simulink model "Torquecontrol_2MW"  (R2020a)
settings: Solver=VariableStepAuto  StartTime=0.0  StopTime=120  RelTol=1e-3  EnableMultiTasking=on
values from neighbouring files (symbols this model uses):
  a1 = 0.5176    [data.mat]
  a2 = 116    [data.mat]
  a3 = 0.4    [data.mat]
  a4 = 5    [data.mat]
  a5 = 21    [data.mat]
  a6 = 0.0068    [data.mat]
  a7 = 0.09    [data.mat]
  a8 = 0.035    [data.mat]
  Ad = 6031.85789489    [data.mat]
  denp = den_P    [Wind_Turbine_Pitch.m]    (also in data.mat = [91260000000000 145900000000000 1.431e+17 7.554e+15 2.279e+1)
  dent = den_P    [Wind_Turbine_Pitch.m]    (also in data.mat = [91260000000000 145900000000000 1.431e+17 7.554e+15 2.279e+1)
  nump = num_P    [Wind_Turbine_Pitch.m]    (also in data.mat = [16590000 26450000 25540000000 6335000000 3680000000000])
  numt = num_T    [Wind_Turbine_Pitch.m]    (also in data.mat = [-75000000 -527900000000 -306700000000000])
  sigma = 1 - Lm^2/(Ls*Lr)    (= 0.0661284179513)    [Generator_specs.m]    (also in data.mat = 0.075)
  Tie = 1    [data.mat]
  Tiu = 10000    [data.mat]
  Tix = 1    [data.mat]
  Tpe = 1    [data.mat]
  Tpu = 10000    [data.mat]
  Tpx = 10000    [data.mat]
undefined symbols (not defined in the file or in its folder): sigbuilder_block
settings Model: Creator=likhi  LastModifiedBy=param
settings DataIOCC: ReturnWorkspaceOutputs=off
settings OptimizationCC: LifeSpan=inf
settings DebuggingCC: SFUnexpectedBacktrackingDiag=warning  SFNoUnconditionalDefaultTransitionDiag=warning  SFExecutionAtInitializationDiag=none  ArithmeticOperatorsInVariantConditions=warning
settings SFSimCC: SimUseLocalCustomCode=off  CustomCodeUndefinedFunction=UseInterfaceOnly
settings RTWCC: RTWUseLocalCustomCode=off
settings CodeAppCC: StateflowObjectComments=on
settings GRTTargetCC: TargetLangStandard=C89/C90 (ANSI)
settings ConfigComp: CovMetricSettings=dw  CovHtmlReporting=on  CovSaveCumulativeToWorkspaceVar=on  CovSaveSingleToWorkspaceVar=on  CovExternalEMLEnable=off

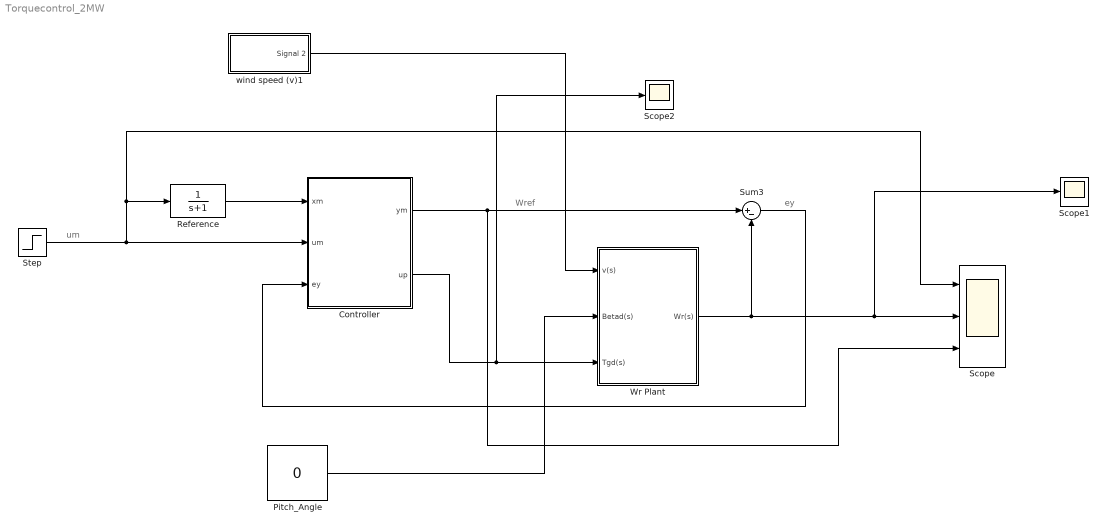
== system Torquecontrol_2MW ==
  note: um
  note: ey
  note: Wref
  Controller : Subsystem
  Pitch_Angle : Constant  Value=0
  Reference : TransferFcn  Denominator=[1 1]
  Scope : Scope  NumInputPorts=3
  Scope1 : Scope
  Scope2 : Scope
  Step : Step  Time=0  After=2  SampleTime=0
  Sum3 : Sum  Inputs=|+-
  Wr Plant : Subsystem
  wind speed (v)1 : Subsystem  Tag=STV Subsys  LoadFcn=sigbuilder_block('load');  StartFcn=sigbuilder_block('start');  StopFcn=sigbuilder_block('stop');  ClipboardFcn=sigbuilder_block('clipboard');  mask(Sigbuilder block){tuvar=[0:10]}
      mask help: Simulink:masks:SigbuilderBlock_MD
      mask init:
      | if ~strcmp(get_param(bdroot(gcbh),'SimulationStatus'),'stopped') tuvar = sigbuilder_block('maskInit'); end
      settings: CopyFcn=sigbuilder_block('copy');  DeleteFcn=sigbuilder_block('delete');  ModelCloseFcn=sigbuilder_block('modelClose');  PreSaveFcn=sigbuilder_block('preSave');  PauseFcn=sigbuilder_block('pause');  ContinueFcn=sigbuilder_block('continue');  NameChangeFcn=sigbuilder_block('namechange');  OpenFcn=sigbuilder_block('open',[6 0 1012.5 477.75 ]);  CloseFcn=sigbuilder_block('close');
      mask Display: plot(0, 0, 100, 100,[2, 2, 32, 32, 2], [68, 8, 8, 68, 68],[32, 2], [38, 38], [32, 19, 2],[53, 60, 44], [32, 17, 17, 2],[16, 16, 31, 31]);txt = getActiveGroup(gcbh);text(2, 100, txt,'verticalAlignment', 'top');
  wires:
  Wr Plant/1(Wr(s)) -> Scope1/1, Scope/2, Sum3/2
  wind speed (v)1/1(Signal 2) -> Wr Plant/1(v(s))
  Sum3/1 -> Controller/3(ey)
  Reference/1 -> Controller/1(xm)
  Step/1 -> Scope/1, Reference/1, Controller/2(um)
  Controller/1(ym) -> Scope/3, Sum3/1
  Pitch_Angle/1 -> Wr Plant/2(Betad(s))
  Controller/2(up) -> Scope2/1, Wr Plant/3(Tgd(s))

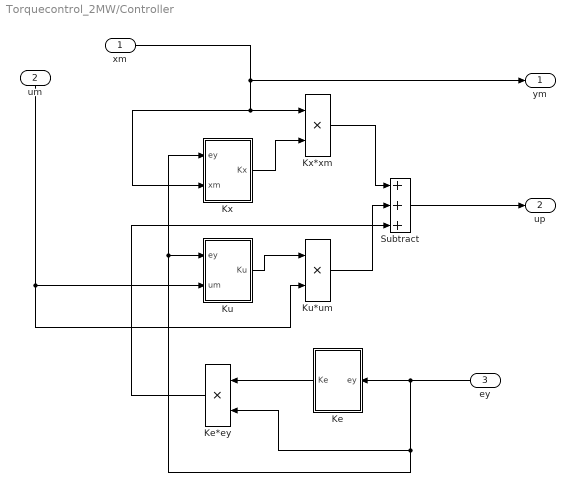
== system Torquecontrol_2MW/Controller ==
  xm : Inport
  um : Inport  Port=2
  ey : Inport  Port=3
  Ke : Subsystem
  Ke*ey : Product
  Ku : Subsystem
  Ku*um : Product
  Kx : Subsystem
  Kx*xm : Product
  Subtract : Sum  Inputs=+++
  ym : Outport
  up : Outport  Port=2
  wires:
  Kx/1(Kx) -> Kx*xm/2
  Ke/1(Ke) -> Ke*ey/1
  Ku*um/1 -> Subtract/2
  Kx*xm/1 -> Subtract/1
  xm/1 -> Kx*xm/1, Kx/2(xm), ym/1
  ey/1 -> Kx/1(ey), Ku/1(ey), Ke*ey/2, Ke/1(ey)
  Ku/1(Ku) -> Ku*um/1
  Ke*ey/1 -> Subtract/3
  um/1 -> Ku/2(um), Ku*um/2
  Subtract/1 -> up/1

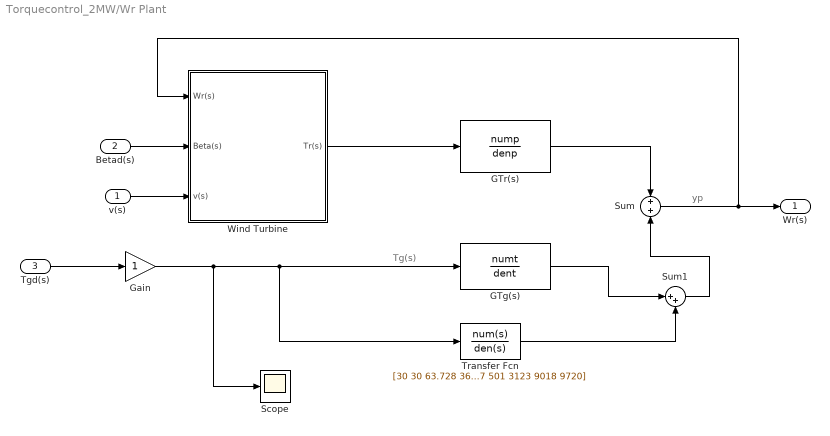
== system Torquecontrol_2MW/Wr Plant ==
  note: yp
  note: Tg(s)
  v(s) : Inport
  Betad(s) : Inport  Port=2
  Tgd(s) : Inport  Port=3
  GTg(s) : TransferFcn  Numerator=numt  Denominator=dent
  GTr(s) : TransferFcn  Numerator=nump  Denominator=denp
  Gain : Gain
  Scope : Scope
  Sum : Sum
  Sum1 : Sum  Inputs=|++
  Transfer Fcn : TransferFcn  Numerator=[30 30 63.728 36.973 30]  Denominator=[1 37 501 3123 9018 9720]
  Wind Turbine : Subsystem  AncestorBlock=re_lib/Wind Generation/Wind Turbine  DialogController=POWERSYS.PowerSysDialog  mask(Wind Turbine){Pnom=2e6, Pelec_base=2e6/0.9, wind_base=9, P_wind_base=0.73, speed_nom=1.2, pitch_angle=0, c1_c6=[0.51763          116          0.4            5           21     0.006795], cp_nom=0.48, lambda_nom=8.1}
      mask prompts: Pnom "Nominal mechanical output power (W):"; Pelec_base "Base power of the electrical generator (VA):"; wind_base "Base wind speed (m/s):"; P_wind_base "Maximum power at base wind speed (pu of nominal mechanical power):"; speed_nom "Base rotational speed (p.u. of base generator speed):"; pitch_angle "Pitch angle beta to display wind-turbine power characteristics (beta >=0)  (deg):"
      mask help:
      | This block implements a variable pitch wind turbine model. The performance coefficient Cp of the turbine is the mechanical output power of the turbine divided by wind power and a function of wind speed, rotational speed, and pitch angle (beta). Cp reaches its maximum value at zero beta. Select the wind-turbine power characteristics display to plot the turbine characteristics at the specified pitch angle.
      |
      | The first input is the generator speed in per unit of the generator base speed. For a synchronous or asynchronous generator, the base speed is the synchronous speed. For a permanent-magnet generator, the base speed is defined as the speed producing nominal voltage at  no load. The second input is the blade pitch angle (beta) in degrees. The third input is the wind speed in m/s.
      |
      | The output is the torque applied to the generator shaft in per unit of the generator ratings.
      |
      | The turbine inertia must be added to the generator inertia.
      mask init:
      | c1=c1_c6(1);c2=c1_c6(2);c3=c1_c6(3);c4=c1_c6(4);c5=c1_c6(5);c6=c1_c6(6);
      | power_initmask();
      mask Help: helpview(psbhelp);
      mask DialogControl DisplayTurbChar Prompt: Display wind turbine power characteristics
      mask DialogControl DisplayTurbChar Callback: WindTurbinePlot(gcb)
      mask Display: disp('');
  Wr(s) : Outport
  wires:
  v(s)/1 -> Wind Turbine/3(v(s))
  Sum/1 -> Wind Turbine/1(Wr(s)), Wr(s)/1
  Tgd(s)/1 -> Gain/1
  GTr(s)/1 -> Sum/1
  Betad(s)/1 -> Wind Turbine/2(Beta(s))
  Wind Turbine/1(Tr(s)) -> GTr(s)/1
  GTg(s)/1 -> Sum1/1
  Transfer Fcn/1 -> Sum1/2
  Sum1/1 -> Sum/2
  Gain/1 -> Scope/1, Transfer Fcn/1, GTg(s)/1

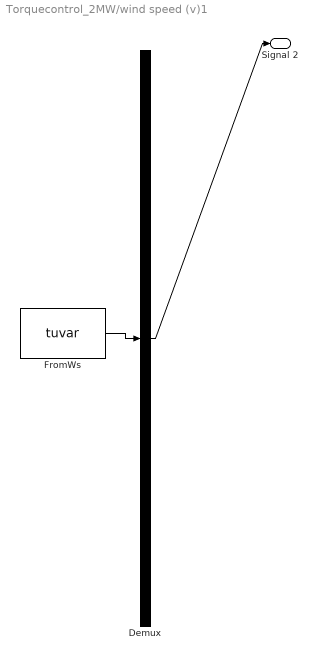
== system Torquecontrol_2MW/wind speed (v)1 ==
  Demux : Demux  Tag=STV Demux  Outputs=1
      settings: DisplayOption=none
  FromWs : FromWorkspace  Tag=STV FromWs  VariableName=tuvar
      SigBuilderData=|
      | common.afterFinalStr = 'Extrapolate'
      | common.sampleTime = 0
      | dataSet(1).timeRange = [0 120]
      | dataSet(1).name = 'Group 1'
      | dataSet(2).timeRange = [0 120]
      | dataSet(2).name = 'Group 2'
      | sbobj.Groups(1).Name = 'Group 1'
      | sbobj.Groups(1).Signals.Name = 'Signal 2'
      | sbobj.Groups(1).Signals.XData = [0 0.1 0.2 0.3 0.4 0.5 0.6 0.7 0.8 0.9 1 1.1 ... (1201 elements, 1x1201)]
      | sbobj.Groups(1).Signals.YData = [15.5376671395 16.8338850146 12.741153139 15.8621733204 15.3187652399 13.6923117037 14.5664079777 15.3426244665 18.5783969397 17.7694370299 13.6501130598 18.0349234663 ... (1201 elements, 1x1201)]
      | sbobj.Groups(1).TimeRange = [0 120]
      | sbobj.Groups(2).Name = 'Group 2'
      | sbobj.Groups(2).Signals.Name = 'Signal 2'
      | sbobj.Groups(2).Signals.XData = [0 1 2 3 4 5 6 7 8 9 10 11 12 13 14 15 16 17 18 19 20 21 22 23 24 25 26 27 28 29 30 31 32 33 34 35 36 37 38 39 40 41 42 43 44 45 46 47 48 49 50 51 52 53 54 55 56 57 58 59 60 61 62 63 64 65 66 67 68 69 70 71 72 73 74 75 76 77 78 79 80 81 82 83 84 85 86 87 88 89 90 91 92 93 94 95 96 97 98 99 100 101 102 103 104 105 106 107 108 109 110 111 112 113 114 115 116 117 118 119 120]
      | sbobj.Groups(2).Signals.YData = [6.01807011575 8.53111911749 8.37266970097 6.38788209314 6.03326297745 6.7836046006 6.68391753827 8.38531742797 6.65170467526 8.20551098078 8.2372434827 9.51972353887 6.62054986454 6.52473145914 8.67572534733 6.26163099795 5.18449703008 7.08672831708 7.50025750546 6.63701916975 6.64930795179 5.63709007085 8.72280393054 7.20137215133 6.45231320782 7.40181236393 7.8343950088 5.95170328812 7.22526321009 6.51763027044 8.65071534952 7.1589257508 5.87531461923 6.88893652325 7.44905097876 9.10058337566 7.03956746808 7.5715725811 8.2007261515 7.50877197187 6.13023828926 6.83893544572 6.34217505374 7.70675183542 8.54031716106 6.97805835356 8.05476174338 6.30324217777 7.15930139 6.82352986481 8.63025921041 7.29396392303 7.76771316613 6.65881339337 6.36659735978 7.39470297405 6.18156140346 5.63827031704 6.69788260596 8.59917448056 6.60767889589 7.22082844093 6.40627813759 4.94960707642 7.00042709296 8.69365989635 6.66847169633 5.84985543786 6.00932777576 7.36418987362 6.57966870551 7.98362168542 6.72423482213 4.91447611455 6.5605287362 7.71192447178 8.02647611247 8.28493457593 8.0007203094 8.07339134627 8.89403249947 8.53443238039 7.17558857287 6.52388222946 6.72025139973 7.70263035474 8.20817483441 6.75244069605 8.51267048749 6.27505286867 6.53466887118 6.61304912341 6.33804960379 7.86990128763 6.81291409702 8.85153725956 6.99387147367 8.86628025483 4.5700315725 7.36181676324 7.28348347922 8.9351889634 7.26172399751 8.77916155129 8.89273585112 6.3796842285 5.80934335084 7.8581940134 6.18492300645 6.8428468059 6.42877121807 7.10081065657 7.59642491901 7.7122037583 7.13564133138 6.05309134985 6.15307228787 7.29230275836 4.8156990126 5.82555531806 5.4342312069]
      | sbobj.Groups(2).TimeRange = [0 120]
  Signal 2 : Outport  Tag=STV Outport
  wires:
  Demux/1 -> Signal 2/1
  FromWs/1 -> Demux/1

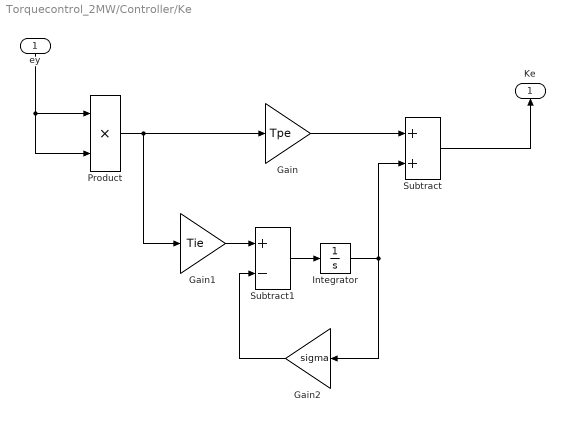
== system Torquecontrol_2MW/Controller/Ke ==
  ey : Inport
  Gain : Gain  Gain=Tpe
  Gain1 : Gain  Gain=Tie
  Gain2 : Gain  Gain=sigma
  Integrator : Integrator
  Product : Product
  Subtract : Sum
  Subtract1 : Sum  Inputs=+-
  Ke : Outport
  wires:
  Subtract/1 -> Ke/1
  ey/1 -> Product/2, Product/1
  Product/1 -> Gain1/1, Gain/1
  Gain/1 -> Subtract/1
  Gain1/1 -> Subtract1/1
  Subtract1/1 -> Integrator/1
  Integrator/1 -> Gain2/1, Subtract/2
  Gain2/1 -> Subtract1/2

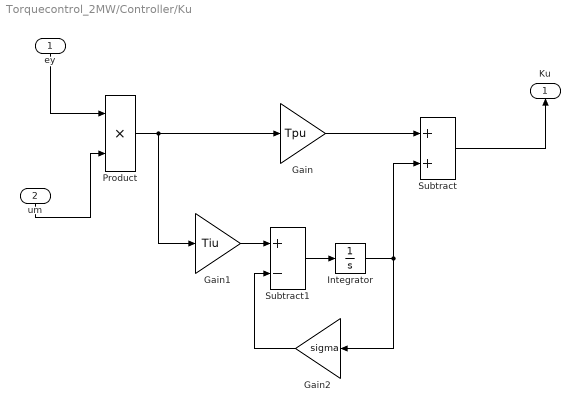
== system Torquecontrol_2MW/Controller/Ku ==
  ey : Inport
  um : Inport  Port=2
  Gain : Gain  Gain=Tpu
  Gain1 : Gain  Gain=Tiu
  Gain2 : Gain  Gain=sigma
  Integrator : Integrator
  Product : Product
  Subtract : Sum
  Subtract1 : Sum  Inputs=+-
  Ku : Outport
  wires:
  Gain2/1 -> Subtract1/2
  Integrator/1 -> Subtract/2, Gain2/1
  Subtract1/1 -> Integrator/1
  Gain1/1 -> Subtract1/1
  Gain/1 -> Subtract/1
  Product/1 -> Gain/1, Gain1/1
  Subtract/1 -> Ku/1
  ey/1 -> Product/1
  um/1 -> Product/2

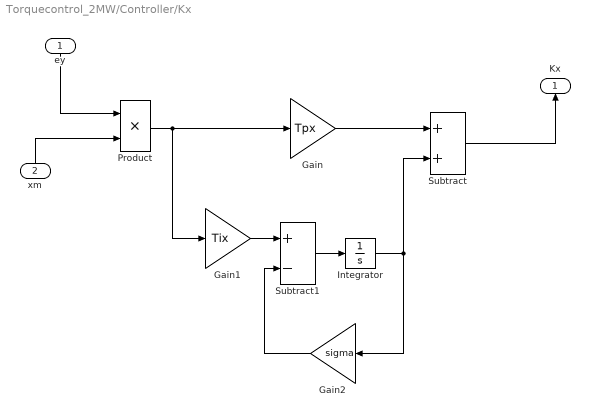
== system Torquecontrol_2MW/Controller/Kx ==
  ey : Inport
  xm : Inport  Port=2
  Gain : Gain  Gain=Tpx
  Gain1 : Gain  Gain=Tix
  Gain2 : Gain  Gain=sigma
  Integrator : Integrator
  Product : Product
  Subtract : Sum
  Subtract1 : Sum  Inputs=+-
  Kx : Outport
  wires:
  Subtract/1 -> Kx/1
  Gain/1 -> Subtract/1
  Gain1/1 -> Subtract1/1
  Subtract1/1 -> Integrator/1
  Integrator/1 -> Gain2/1, Subtract/2
  Gain2/1 -> Subtract1/2
  Product/1 -> Gain1/1, Gain/1
  ey/1 -> Product/1
  xm/1 -> Product/2

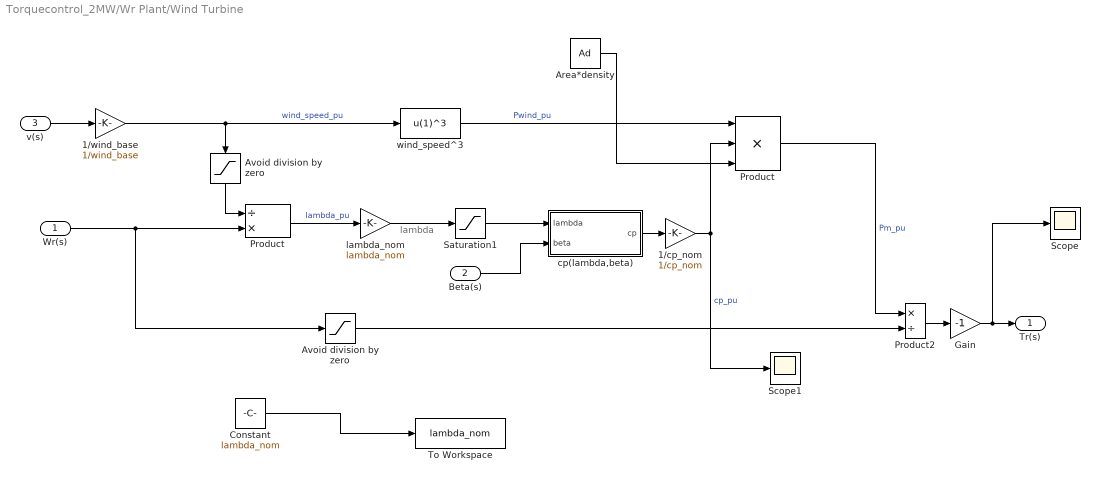
== system Torquecontrol_2MW/Wr Plant/Wind Turbine ==
  note: lambda
  Wr(s) : Inport
  Beta(s) : Inport  Port=2
  v(s) : Inport  Port=3
  1/cp_nom : Gain  Gain=1/cp_nom  SaturateOnIntegerOverflow=on  OutDataTypeStr=Inherit: Same as input  ParamDataTypeStr=Inherit: Same as input
  1/wind_base : Gain  Gain=1/wind_base  SaturateOnIntegerOverflow=on  OutDataTypeStr=Inherit: Same as input  ParamDataTypeStr=Inherit: Same as input
  Area*density : Constant  Value=Ad
  Avoid division by zero : Saturate  UpperLimit=1e6  LowerLimit=1e-6
  "Avoid division by zero " : Saturate  UpperLimit=1e6  LowerLimit=1e-6
  Constant : Constant  Value=lambda_nom
  Gain : Gain  Gain=-1  SaturateOnIntegerOverflow=on  OutDataTypeStr=Inherit: Same as input  ParamDataTypeStr=Inherit: Same as input
  Product : Product  Inputs=/*  SaturateOnIntegerOverflow=on  OutDataTypeStr=Inherit: Same as first input
  "Product " : Product  Inputs=3  SaturateOnIntegerOverflow=on  OutDataTypeStr=Inherit: Same as first input
  Product2 : Product  Inputs=*/  InputSameDT=on  SaturateOnIntegerOverflow=on  OutDataTypeStr=Inherit: Same as first input
  Saturation1 : Saturate  UpperLimit=inf  LowerLimit=1e-6
  Scope : Scope
  Scope1 : Scope
  To Workspace : ToWorkspace  VariableName=lambda_nom  SaveFormat=Timeseries  SampleTime=-1
  cp(lambda,beta) : Subsystem
  lambda_nom : Gain  Gain=lambda_nom  SaturateOnIntegerOverflow=on  OutDataTypeStr=Inherit: Same as input  ParamDataTypeStr=Inherit: Same as input
  wind_speed^3 : Fcn  Expr=u(1)^3
  Tr(s) : Outport
  wires:
  Area*density/1 -> "Product "/3
  Wr(s)/1 -> Avoid division by zero/1, Product/2
  "Avoid division by zero "/1 -> Product/1
  1/wind_base/1 -> "Avoid division by zero "/1, wind_speed^3/1  "wind_speed_pu"
  Product/1 -> lambda_nom/1  "lambda_pu"
  Saturation1/1 -> cp(lambda,beta)/1(lambda)
  1/cp_nom/1 -> "Product "/2, Scope1/1  "cp_pu"
  lambda_nom/1 -> Saturation1/1
  "Product "/1 -> Product2/1  "Pm_pu"
  v(s)/1 -> 1/wind_base/1
  Avoid division by zero/1 -> Product2/2
  Product2/1 -> Gain/1
  wind_speed^3/1 -> "Product "/1  "Pwind_pu"
  cp(lambda,beta)/1(cp) -> 1/cp_nom/1
  Beta(s)/1 -> cp(lambda,beta)/2(beta)
  Gain/1 -> Scope/1, Tr(s)/1
  Constant/1 -> To Workspace/1

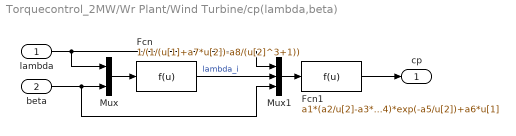
== system Torquecontrol_2MW/Wr Plant/Wind Turbine/cp(lambda,beta) ==
  lambda : Inport
  beta : Inport  Port=2
  Fcn : Fcn  Expr=1/(1/(u[1]+a7*u[2])-a8/(u[2]^3+1))
  Fcn1 : Fcn  Expr=a1*(a2/u[2]-a3*u[3]-a4)*exp(-a5/u[2])+a6*u[1]
  Mux : Mux  Inputs=2
  Mux1 : Mux  Inputs=3
  cp : Outport
  wires:
  Mux/1 -> Fcn/1
  beta/1 -> Mux/2, Mux1/3
  Mux1/1 -> Fcn1/1
  lambda/1 -> Mux/1, Mux1/1
  Fcn1/1 -> cp/1
  Fcn/1 -> Mux1/2  "lambda_i"
